simulink model "controlScheme_UDP_3Beads"  (R2019b)
settings: Solver=FixedStepDiscrete  StartTime=0.0  StopTime=Inf  FixedStep=1/30  RelTol=1e-3
InitFcn:
  | tb = twinbeam('147.32.86.177', 30000);
  | img = tb.get();
  | f = figure(25)
  | imshow(img);
  | 
  | tb.tracker_init(3);
  | pause(2)
  | 
  | tb.coords_subs(30006);
  | pause(1)
  | 
  | close(f)
StopFcn:
  | delete(tb);
  | 
  | gen_udp = udp('147.32.86.177', 30001);
  | fopen(gen_udp);
  | fwrite(gen_udp, uint8('d'));
  | fclose(gen_udp);
  | delete(gen_udp);
model workspace (MAT data in the model file):
  NumberOfBeads = Simulink.Parameter
  NumberOfBeads.Value = 1
  NumberOfBeads.DataType = 'auto'
  NumberOfBeads.Dimensions = [1 1]
undefined symbols (not defined in the file): DiscIntNeverNeededParam, H, Joystick, N_objs, Standard_Devices, UDP_Protocol
libraries: sldrtlib x4, instrumentlib x1
settings Model: SimulationMode=accelerator  EnablePacing=on  ParameterArgumentNames=NumberOfBeads  OrderedModelArguments=off  Creator=marti  LastModifiedBy=marti
settings SolverCC: MinimalZcImpactIntegration=on
settings DebuggingCC: ReadBeforeWriteMsg=DisableAll  WriteAfterWriteMsg=DisableAll  WriteAfterReadMsg=DisableAll  MultiTaskDSMMsg=none
settings ModelReferenceCC: UpdateModelReferenceTargets=IfOutOfDate
settings SFSimCC: SFSimEcho=off
settings RTWCC: Description=Simulink Desktop Real-Time  SystemTargetFile=sldrt.tlc  TemplateMakefile=sldrt.tmf  RTWCompilerOptimization=on
settings CodeAppCC: MaxIdLength=95
settings SimulinkDesktopRealTimeCC: TargetPreCompLibLocation=C:\Program Files\MATLAB\R2019b\toolbox\sldrt\lib\win64  PreserveStateflowLocalDataDimensions=off

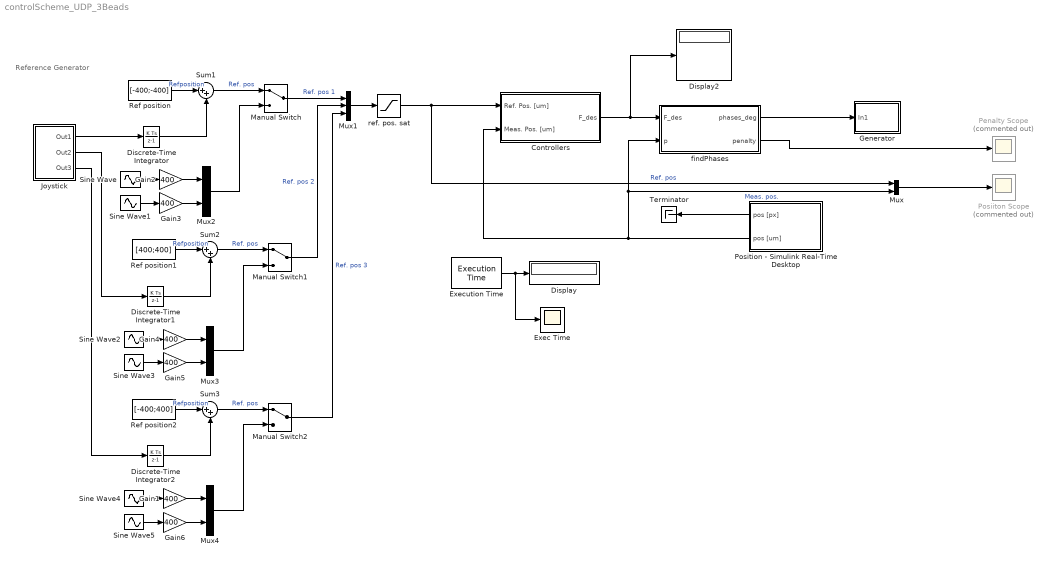
== system controlScheme_UDP_3Beads ==
  note: Reference Generator
  Controllers : Subsystem  mask{P_const=300e-14, F_max=30e-11}
      mask prompts: P_const "P constant"; F_max "F max"
  Discrete-Time Integrator : DiscreteIntegrator  gainval=1  SampleTime=-1  ICPrevOutput=DiscIntNeverNeededParam  ICPrevScaledInput=DiscIntNeverNeededParam
  Discrete-Time Integrator1 : DiscreteIntegrator  gainval=1  SampleTime=-1  ICPrevOutput=DiscIntNeverNeededParam  ICPrevScaledInput=DiscIntNeverNeededParam
  Discrete-Time Integrator2 : DiscreteIntegrator  gainval=1  SampleTime=-1  ICPrevOutput=DiscIntNeverNeededParam  ICPrevScaledInput=DiscIntNeverNeededParam
  Display : Display
  Display2 : Display
  Exec Time : Scope
  Execution Time : sldrtlib/Target Profiling/Execution Time  ShowTaskTimes=off
      settings: SourceProductBaseCode=WT
  Gain{1..6} (6 alike) : Gain  Gain=400
  Generator : Subsystem
  Joystick : Subsystem
  Manual Switch : ManualSwitch
  Manual Switch1 : ManualSwitch
  Manual Switch2 : ManualSwitch
  Mux{,2..4} (4 alike) : Mux  Inputs=2
  Mux1 : Mux  Inputs=3
  Penalty Scope : Scope  Commented=on
  Posiiton Scope : Scope  Commented=on
  Position - Simulink Real-Time Desktop : Subsystem  VariantControl=(default)  mask{N_objs=3}
      mask prompts: N_objs "Number of objects"
  Ref position : Constant  Value=[-400;-400]
  Ref position1 : Constant  Value=[400;400]
  Ref position2 : Constant  Value=[-400;400]
  Sine Wave : Sin  Frequency=2*pi/40  SampleTime=0
  Sine Wave1 : Sin  Frequency=2*pi/20  Phase=-pi  SampleTime=0
  Sine Wave2 : Sin  Frequency=2*pi/40  Phase=2*pi/3  SampleTime=0
  Sine Wave3 : Sin  Frequency=2*pi/20  Phase=-pi + 2*pi/3  SampleTime=0
  Sine Wave4 : Sin  Frequency=2*pi/40  Phase=2*2*pi/3  SampleTime=0
  Sine Wave5 : Sin  Frequency=2*pi/20  Phase=-pi + 2*2*pi/3  SampleTime=0
  Sum1 : Sum  Inputs=|++
  Sum2 : Sum  Inputs=|++
  Sum3 : Sum  Inputs=|++
  Terminator : Terminator
  findPhases : MATLAB Function  TreatAsAtomicUnit=on
  ref. pos. sat : Saturate  UpperLimit=600  LowerLimit=-600
  wires:
  Controllers/1(F_des) -> Display2/1, findPhases/1(F_des)
  Position - Simulink Real-Time Desktop/2(pos [um]) -> Mux/2, findPhases/2(p), Controllers/2(Meas. Pos. [um])  "Meas. pos."
  Execution Time/1 -> Exec Time/1, Display/1
  findPhases/1(phases_deg) -> Generator/1(In1)
  findPhases/2(penalty) -> Penalty Scope/1
  Mux/1 -> Posiiton Scope/1
  Position - Simulink Real-Time Desktop/1(pos [px]) -> Terminator/1
  ref. pos. sat/1 -> Mux/1, Controllers/1(Ref. Pos. [um])  "Ref. pos"
  Manual Switch2/1 -> Mux1/3  "Ref. pos 3"
  Sine Wave1/1 -> Gain3/1
  Ref position2/1 -> Sum3/1  "Refposition"
  Gain5/1 -> Mux3/2
  Gain6/1 -> Mux4/2
  Joystick/3(Out3) -> Discrete-Time Integrator2/1
  Sine Wave5/1 -> Gain6/1
  Sine Wave4/1 -> Gain1/1
  Joystick/2(Out2) -> Discrete-Time Integrator1/1
  Sum3/1 -> Manual Switch2/1  "Ref. pos"
  Sum2/1 -> Manual Switch1/1  "Ref. pos"
  Discrete-Time Integrator2/1 -> Sum3/2
  Ref position1/1 -> Sum2/1  "Refposition"
  Manual Switch1/1 -> Mux1/2  "Ref. pos 2"
  Mux4/1 -> Manual Switch2/2
  Sine Wave2/1 -> Gain4/1
  Sum1/1 -> Manual Switch/1  "Ref. pos"
  Ref position/1 -> Sum1/1  "Refposition"
  Sine Wave3/1 -> Gain5/1
  Mux1/1 -> ref. pos. sat/1
  Gain4/1 -> Mux3/1
  Mux3/1 -> Manual Switch1/2
  Gain3/1 -> Mux2/2
  Discrete-Time Integrator/1 -> Sum1/2
  Sine Wave/1 -> Gain2/1
  Gain2/1 -> Mux2/1
  Mux2/1 -> Manual Switch/2
  Manual Switch/1 -> Mux1/1  "Ref. pos 1"
  Joystick/1(Out1) -> Discrete-Time Integrator/1
  Discrete-Time Integrator1/1 -> Sum2/2
  Gain1/1 -> Mux4/1

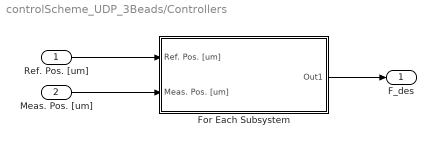
== system controlScheme_UDP_3Beads/Controllers ==
  Ref. Pos. [um] : Inport
  Meas. Pos. [um] : Inport  Port=2
  For Each Subsystem : Subsystem  TreatAsAtomicUnit=on
  F_des : Outport
  wires:
  Ref. Pos. [um]/1 -> For Each Subsystem/1(Ref. Pos. [um])
  For Each Subsystem/1(Out1) -> F_des/1
  Meas. Pos. [um]/1 -> For Each Subsystem/2(Meas. Pos. [um])

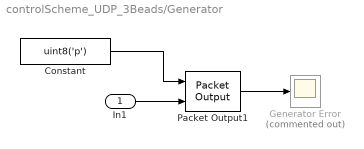
== system controlScheme_UDP_3Beads/Generator ==
  In1 : Inport
  Constant : Constant  Value=uint8('p')
  Generator Error : Scope  Commented=on
  Packet Output1 : sldrtlib/Packet Output  SampleTime=1/30  MaxMissedTicks=200  ShowMissedTicks=off  YieldWhenWaiting=off  DrvName=Standard_Devices/UDP_Protocol  DrvAddress=30001  DrvOptions=[0 30001 49 52 55 46 51 50 46 56 54 46 49 55 55 0 0 0 0 0 0 0 0 0 0 0 0 0 0 0 0 0 0 0 0 0 0 0 0 0 0 0 0 0 0 0 0 0 0 0 0 0 0 0 0 0 0 0 0 0 0 0 0 0 0 0 0 0 0 0 0 0 0 0 0 0 0 0 0 0 0 0 0 0 0 0 0 0 0 0 0 0 0 0 0 0 0 0 0 0 0 0 0 0 0 0 0 0 0 0 0 0 0 0 0 0 0 0 0 0 0 0 0 0 0 0 0 0 0 0 0 0 0 0 0 0 0 0 0 0 0 0 0 0 0 0 0 0 0 0 0 0 0 0 0 0 0 0 0 0 0 0 0 0 0 0 0 0 0 0 0 0 0 0 0 0 0 0 0 0 0 0 0 0 0 0 0 0 0 0 0 0 0 0 0 0 0 0 0 0 0 0 0 0 0 0 0 0 0 0 0 0 0 0 0 0 0 0 0 0 0 0 0 0 0 0 0 0 0 0 0 0 0 0 0 0 0 0 0 0 0 0 0 0 0 0 0 0 0 0 0 0 0 0 0 0]  PacketSize=56*2+1  DataTypes={'uint8', '56*uint16'}  ShowReady=off  ShowError=on  PacketID=1  ByteOrder=1  InitialValue=[]  FinalValue=[]
      settings: AttributesFormatString=UDP Protocol [30001]
  wires:
  In1/1 -> Packet Output1/2
  Packet Output1/1 -> Generator Error/1
  Constant/1 -> Packet Output1/1

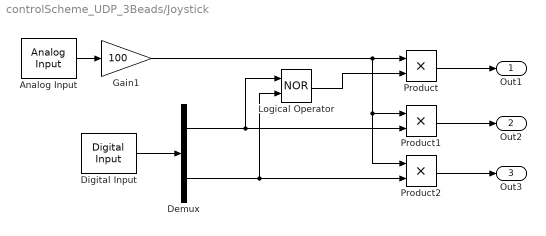
== system controlScheme_UDP_3Beads/Joystick ==
  Analog Input : sldrtlib/Analog Input  SampleTime=0.1  MaxMissedTicks=200  ShowMissedTicks=off  YieldWhenWaiting=off  DrvName=Standard_Devices/Joystick  DrvAddress=1  DrvOptions=zeros(1,0)  Channels=[1:2]  RangeMode=1  VoltRange=1  DataType=1
      settings: AttributesFormatString=Joystick [1]
  Demux : Demux  Outputs=2
  Digital Input : sldrtlib/Digital Input  SampleTime=0.1  MaxMissedTicks=100  ShowMissedTicks=off  YieldWhenWaiting=off  DrvName=Standard_Devices/Joystick  DrvAddress=1  DrvOptions=zeros(1,0)  Channels=1:(N_objs-1)  BitMode=1  DataType=9
      settings: AttributesFormatString=Joystick [1]  SourceProductBaseCode=WT
  Gain1 : Gain  Gain=100
  Logical Operator : Logic  Operator=NOR  AllPortsSameDT=off  OutDataTypeStr=boolean
  Product : Product
  Product1 : Product
  Product2 : Product
  Out1 : Outport
  Out2 : Outport  Port=2
  Out3 : Outport  Port=3
  wires:
  Product1/1 -> Out2/1
  Logical Operator/1 -> Product/2
  Product/1 -> Out1/1
  Demux/1 -> Logical Operator/1, Product1/2
  Analog Input/1 -> Gain1/1
  Gain1/1 -> Product/1, Product2/1, Product1/1
  Digital Input/1 -> Demux/1
  Demux/2 -> Logical Operator/2, Product2/2
  Product2/1 -> Out3/1

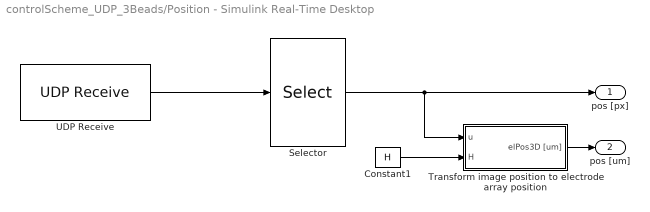
== system controlScheme_UDP_3Beads/Position - Simulink Real-Time Desktop ==
  Constant1 : Constant  Value=H
  Selector : Selector  InputPortWidth=8  IndexOptions=Index vector (dialog)  Indices=[3:8]  OutputSizes=1
  Transform image position to electrode array position : Subsystem  TreatAsAtomicUnit=on
  UDP Receive : instrumentlib/UDP Receive  Host=147.32.86.177  Port=30006  LocalPort=30006  EnablePortSharing=off  GetLatestData=on  DataSize="[2+2*N_objs  1]"  DataType=uint16  ASCIIFormatting=%f,  Terminator=LF  ByteOrder=LittleEndian  EnableBlockingMode=on  Timeout=1  SampleTime=-1  LocalAddress=0.0.0.0
  pos [px] : Outport
  pos [um] : Outport  Port=2  Unit=um
  wires:
  Transform image position to electrode array position/1(elPos3D [um]) -> pos [um]/1
  Selector/1 -> Transform image position to electrode array position/1(u), pos [px]/1
  Constant1/1 -> Transform image position to electrode array position/2(H)
  UDP Receive/1 -> Selector/1

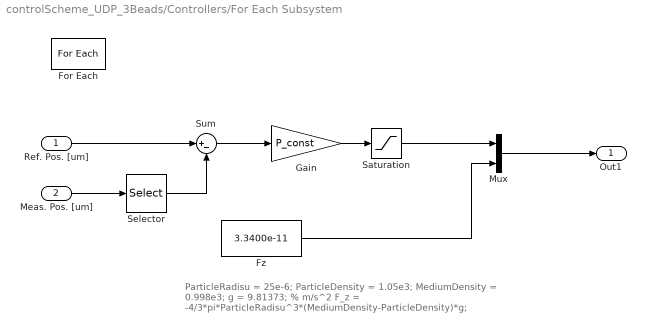
== system controlScheme_UDP_3Beads/Controllers/For Each Subsystem ==
  note: ParticleRadisu = 25e-6;
      | ParticleDensity = 1.05e3;
      | MediumDensity = 0.998e3;
      | g = 9.81373; % m/s^2
      | F_z = -4/3*pi*ParticleRadisu^3*(MediumDensity-ParticleDensity)*g;
  Ref. Pos. [um] : Inport  Partition=on  PartitionDimension=1  PartitionWidth=2  PartitionOffset=0
  Meas. Pos. [um] : Inport  Port=2  Partition=on  PartitionDimension=1  PartitionWidth=3  PartitionOffset=0
  For Each : ForEach  DisableCoverage=on
  Fz : Constant  Value=3.3400e-11
  Gain : Gain  Gain=P_const
  Mux : Mux  Inputs=2
  Saturation : Saturate  UpperLimit=F_max  LowerLimit=-F_max
  Selector : Selector  InputPortWidth=3  IndexOptions=Index vector (dialog)  Indices=[1 2]  OutputSizes=1
  Sum : Sum  Inputs=|+-
  Out1 : Outport  ConcatenationDimension=1
  wires:
  Gain/1 -> Saturation/1
  Mux/1 -> Out1/1
  Saturation/1 -> Mux/1
  Fz/1 -> Mux/2
  Meas. Pos. [um]/1 -> Selector/1
  Sum/1 -> Gain/1
  Selector/1 -> Sum/2
  Ref. Pos. [um]/1 -> Sum/1

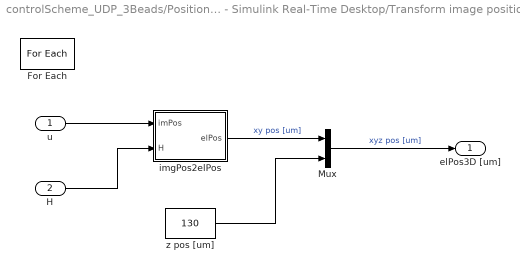
== system controlScheme_UDP_3Beads/Position - Simulink Real-Time Desktop/Transform image position to electrode array position ==
  u : Inport  Partition=on  PartitionDimension=1  PartitionWidth=2  PartitionOffset=0
  H : Inport  Port=2
  For Each : ForEach  DisableCoverage=on
  Mux : Mux  Inputs=2
  imgPos2elPos : MATLAB Function  TreatAsAtomicUnit=on
  z pos [um] : Constant  Value=130
  elPos3D [um] : Outport  ConcatenationDimension=1
  wires:
  H/1 -> imgPos2elPos/2(H)
  u/1 -> imgPos2elPos/1(imPos)
  imgPos2elPos/1(elPos) -> Mux/1  "xy pos [um]"
  Mux/1 -> elPos3D [um]/1  "xyz pos [um]"
  z pos [um]/1 -> Mux/2

== matlab function controlScheme_UDP_3Beads/Position - Simulink Real-Time Desktop/Transform image position to electrode array position/imgPos2elPos ==
  data: imPos input; elPos output; H input
function elPos = fcn(imPos, H)
tmp = H*[double(imPos(2));double(imPos(1));1];
elPos = [tmp(1)/tmp(3); tmp(2)/tmp(3)];

== matlab function controlScheme_UDP_3Beads/findPhases ==
  data: F_des input; p input; phases_deg output; penalty output
function [phases_deg, penalty] = fcn(F_des, p)
[phases_rad, penalty] = findPhasesFoGivenF(p*1e-6, F_des);
phases_deg = rad2deg(phases_rad);
phases_deg = round(mod(phases_deg, 360));
